simulink model "WeatherAPI"  (R2024b)
settings: Solver=VariableStepAuto  StartTime=0.0  StopTime=86400  FixedStep=0.05  RelTol=1e-3
libraries: spsCurrentMeasurementLib x6, spsGroundLib x6, eePowerMeasurement x6, spsPVArrayLib x6, spsSeriesRLCLoadLib x6, spsVoltageMeasurementLib x6, spspowerguiLib x1
settings Model: Creator=mitphanase  LastModifiedBy=DELL
settings RTWCC: GenCodeOnly=on

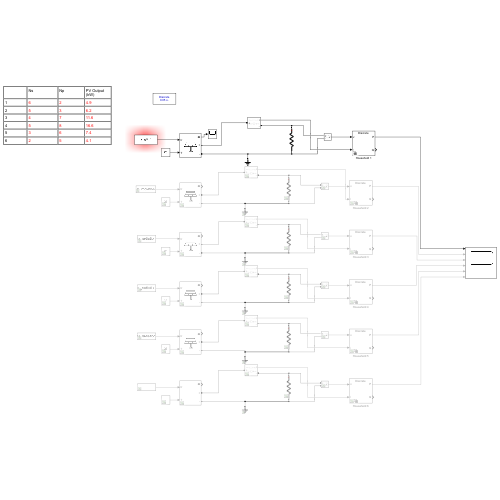
[thumbnail: Simulink's stored preview of the top-level diagram]
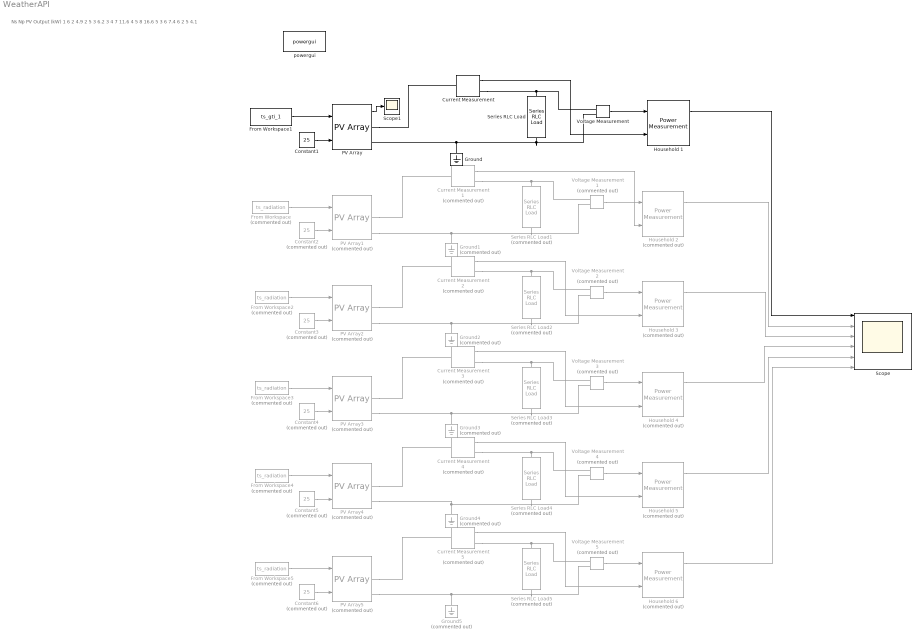
== system WeatherAPI ==
  note: ​
      | Ns
      | Np
      | PV Output (kW)
      |
      | 1
      | 6
      | 2
      | 4.9
      |
      | 2
      | 5
      | 3
      | 6.2
      |
      | 3
      | 4
      | 7
      | 11.6
      |
      | 4
      | 5
      | 8
      | 16.6
      |
      | 5
      | 3
      | 6
      | 7.4
      |
      | 6
      | 2
      | 5
      | 4.1
  Constant1 : Constant  Value=25
  Constant{2..6} (5 alike) : Constant  Commented=on  Value=25
  Current Measurement : spsCurrentMeasurementLib/Current Measurement  PhasorSimulation=off  OutputType=Complex  PSBequivalent=0
  Current Measurement{1..5} (5 alike) : spsCurrentMeasurementLib/Current Measurement  Commented=on  PhasorSimulation=off  OutputType=Complex  PSBequivalent=0
  From Workspace{,2..4} (4 alike) : FromWorkspace  Commented=on  VariableName=ts_radiation  OutDataTypeStr=double
  From Workspace1 : FromWorkspace  VariableName=ts_gti_1  OutDataTypeStr=double
  From Workspace5 : FromWorkspace  Commented=on  VariableName=ts_radiation
  Ground : spsGroundLib/Ground  LConnTagsString=a
  Ground{1..5} (5 alike) : spsGroundLib/Ground  Commented=on  LConnTagsString=a
  Household 1 : eePowerMeasurement/Power Measurement  LabelModeActiveChoice=Discrete  F=60  K=[0]  Ts=60
  "Household 2 " : eePowerMeasurement/Power Measurement  Commented=on  LabelModeActiveChoice=Discrete  F=60  K=[0]  Ts=60
  Household {3..6} (4 alike) : eePowerMeasurement/Power Measurement  Commented=on  LabelModeActiveChoice=Discrete  F=60  K=[0]  Ts=60
  PV Array : spsPVArrayLib/PV Array  Npar=2  Nser=6  PlotType=array @ 1000 W/m2 & specified temperatures  S_vec="[ 1000  500  100 ]"  Temp_C_vec="[ 45 25  ]"  ModuleName=SunPower SPR-415E-WHT-D  PlotWhenSelected=off  Pm=414.801  Ncell=128  Voc=85.3  Isc=6.09  Vm=72.9  Im=5.69  beta_Voc_pc=-0.229  alpha_Isc_pc=0.030706  beta_Voc=-0.19534  alpha_Isc=0.00187  IL=6.0978  I0=7.1698e-13  nI=0.87223  Rsh=419.7781  Rs=0.53711  RobustModel=off  RobustCellTemperature=313.3991  BAL=on  Tc=1e-6  Tfilter=5e-5
  PV Array1 : spsPVArrayLib/PV Array  Commented=on  Npar=3  Nser=5  PlotType=array @ 1000 W/m2 & specified temperatures  S_vec="[ 1000  500  100 ]"  Temp_C_vec="[ 45 25  ]"  ModuleName=SunPower SPR-415E-WHT-D  PlotWhenSelected=off  Pm=414.801  Ncell=128  Voc=85.3  Isc=6.09  Vm=72.9  Im=5.69  beta_Voc_pc=-0.229  alpha_Isc_pc=0.030706  beta_Voc=-0.19534  alpha_Isc=0.00187  IL=6.0978  I0=7.1698e-13  nI=0.87223  Rsh=419.7781  Rs=0.53711  RobustModel=off  RobustCellTemperature=313.3991  BAL=on  Tc=1e-6  Tfilter=5e-5
  PV Array2 : spsPVArrayLib/PV Array  Commented=on  Npar=4  Nser=7  PlotType=array @ 1000 W/m2 & specified temperatures  S_vec="[ 1000  500  100 ]"  Temp_C_vec="[ 45 25  ]"  ModuleName=SunPower SPR-415E-WHT-D  PlotWhenSelected=off  Pm=414.801  Ncell=128  Voc=85.3  Isc=6.09  Vm=72.9  Im=5.69  beta_Voc_pc=-0.229  alpha_Isc_pc=0.030706  beta_Voc=-0.19534  alpha_Isc=0.00187  IL=6.0978  I0=7.1698e-13  nI=0.87223  Rsh=419.7781  Rs=0.53711  RobustModel=off  RobustCellTemperature=313.3991  BAL=on  Tc=1e-6  Tfilter=5e-5
  PV Array3 : spsPVArrayLib/PV Array  Commented=on  Npar=6  Nser=7  PlotType=array @ 1000 W/m2 & specified temperatures  S_vec="[ 1000  500  100 ]"  Temp_C_vec="[ 45 25  ]"  ModuleName=SunPower SPR-415E-WHT-D  PlotWhenSelected=off  Pm=414.801  Ncell=128  Voc=85.3  Isc=6.09  Vm=72.9  Im=5.69  beta_Voc_pc=-0.229  alpha_Isc_pc=0.030706  beta_Voc=-0.19534  alpha_Isc=0.00187  IL=6.0978  I0=7.1698e-13  nI=0.87223  Rsh=419.7781  Rs=0.53711  RobustModel=off  RobustCellTemperature=313.3991  BAL=on  Tc=1e-6  Tfilter=5e-5
  PV Array4 : spsPVArrayLib/PV Array  Commented=on  Npar=3  Nser=6  PlotType=array @ 1000 W/m2 & specified temperatures  S_vec="[ 1000  500  100 ]"  Temp_C_vec="[ 45 25  ]"  ModuleName=SunPower SPR-415E-WHT-D  PlotWhenSelected=off  Pm=414.801  Ncell=128  Voc=85.3  Isc=6.09  Vm=72.9  Im=5.69  beta_Voc_pc=-0.229  alpha_Isc_pc=0.030706  beta_Voc=-0.19534  alpha_Isc=0.00187  IL=6.0978  I0=7.1698e-13  nI=0.87223  Rsh=419.7781  Rs=0.53711  RobustModel=off  RobustCellTemperature=313.3991  BAL=on  Tc=1e-6  Tfilter=5e-5
  PV Array5 : spsPVArrayLib/PV Array  Commented=on  Npar=2  Nser=5  PlotType=array @ 1000 W/m2 & specified temperatures  S_vec="[ 1000  500  100 ]"  Temp_C_vec="[ 45 25  ]"  ModuleName=SunPower SPR-415E-WHT-D  PlotWhenSelected=off  Pm=414.801  Ncell=128  Voc=85.3  Isc=6.09  Vm=72.9  Im=5.69  beta_Voc_pc=-0.229  alpha_Isc_pc=0.030706  beta_Voc=-0.19534  alpha_Isc=0.00187  IL=6.0978  I0=7.1698e-13  nI=0.87223  Rsh=419.7781  Rs=0.53711  RobustModel=off  RobustCellTemperature=313.3991  BAL=on  Tc=1e-6  Tfilter=5e-5
  Scope : Scope  NumInputPorts=6
  Scope1 : Scope
  Series RLC Load : spsSeriesRLCLoadLib/Series RLC Load  LConnTagsString=a  RConnTagsString=__new0  NominalVoltage=400  NominalFrequency=0.0000001  ActivePower=2000  InductivePower=0  CapacitivePower=0  Setx0=off  InitialVoltage=0  SetiL0=off  InitialCurrent=0  Measurements=Branch voltage and current  LoadType=constant I
  Series RLC Load1 : spsSeriesRLCLoadLib/Series RLC Load  Commented=on  LConnTagsString=a  RConnTagsString=__new0  NominalVoltage=400  NominalFrequency=0.0000001  ActivePower=3500  InductivePower=0  CapacitivePower=0  Setx0=off  InitialVoltage=0  SetiL0=off  InitialCurrent=0  Measurements=Branch voltage and current  LoadType=constant I
  Series RLC Load2 : spsSeriesRLCLoadLib/Series RLC Load  Commented=on  LConnTagsString=a  RConnTagsString=__new0  NominalVoltage=400  NominalFrequency=0.0000001  ActivePower=6000  InductivePower=0  CapacitivePower=0  Setx0=off  InitialVoltage=0  SetiL0=off  InitialCurrent=0  Measurements=Branch voltage and current  LoadType=constant I
  Series RLC Load3 : spsSeriesRLCLoadLib/Series RLC Load  Commented=on  LConnTagsString=a  RConnTagsString=__new0  NominalVoltage=400  NominalFrequency=0.0000001  ActivePower=10000  InductivePower=0  CapacitivePower=0  Setx0=off  InitialVoltage=0  SetiL0=off  InitialCurrent=0  Measurements=Branch voltage and current  LoadType=constant I
  Series RLC Load4 : spsSeriesRLCLoadLib/Series RLC Load  Commented=on  LConnTagsString=a  RConnTagsString=__new0  NominalVoltage=400  NominalFrequency=0.0000001  ActivePower=5000  InductivePower=0  CapacitivePower=0  Setx0=off  InitialVoltage=0  SetiL0=off  InitialCurrent=0  Measurements=Branch voltage and current  LoadType=constant I
  Series RLC Load5 : spsSeriesRLCLoadLib/Series RLC Load  Commented=on  LConnTagsString=a  RConnTagsString=__new0  NominalVoltage=400  NominalFrequency=0.0000001  ActivePower=4000  InductivePower=0  CapacitivePower=0  Setx0=off  InitialVoltage=0  SetiL0=off  InitialCurrent=0  Measurements=Branch voltage and current  LoadType=constant I
  Voltage Measurement : spsVoltageMeasurementLib/Voltage Measurement  PhasorSimulation=off  OutputType=Complex  PSBequivalent=0
  Voltage Measurement{1..5} (5 alike) : spsVoltageMeasurementLib/Voltage Measurement  Commented=on  PhasorSimulation=off  OutputType=Complex  PSBequivalent=0
  powergui : spspowerguiLib/powergui  Priority=1  SimulationMode=Discrete  SampleTime=0.05  frequency=60  Iterations=50  frequencyindice=0  Pbase=100e6  ErrMax=1e-4  UnitsV=kV  UnitsW=MW  buscounter=0  FunctionMessages=off  echomessages=off  EnableUseOfTLC=off  CurrentSourceSwitches=off  DisableSnubberDevices=off  DisableRonSwitches=off  DisableVfSwitches=off  DisplayEquations=off  AutomaticDiscreteSolvers=off  SolverType=Tustin/Backward Euler (TBE)  Interpol=off  ExternalGateDelay=off  methode=off  Ts=100  x0status=blocks  SPID=on  SwTol=0  HookPort=off  NonlinearTolerance=1e-4  nMaxIteration=100  ContinueOnMaxIteration=off  RestoreLinks=warning  ResistiveCurrentMeasurement=off  Frange=[0:2:500]  Ylog=off  Xlog=on  ShowGrid=off  save=off  variable=ZData  structure=0  ZoomFFT=off  StartTime=0.0  cycles=1  DisplayStyle=1  fundamental=60  FreqAxis=off  MaxFrequency=1000  frequencyindicesteady=1  RmsSteady=1  display=off
  wires:
  Constant1/1 -> PV Array/2
  From Workspace1/1 -> PV Array/1
  Current Measurement/1 -> Household 1/2
  Voltage Measurement/1 -> Household 1/1
  From Workspace/1 -> PV Array1/1
  From Workspace2/1 -> PV Array2/1
  From Workspace3/1 -> PV Array3/1
  From Workspace4/1 -> PV Array4/1
  From Workspace5/1 -> PV Array5/1
  Constant2/1 -> PV Array1/2
  Constant3/1 -> PV Array2/2
  Constant4/1 -> PV Array3/2
  Constant5/1 -> PV Array4/2
  Constant6/1 -> PV Array5/2
  Current Measurement1/1 -> "Household 2 "/2
  Voltage Measurement1/1 -> "Household 2 "/1
  Current Measurement2/1 -> Household 3/2
  Voltage Measurement2/1 -> Household 3/1
  Current Measurement3/1 -> Household 4/2
  Voltage Measurement3/1 -> Household 4/1
  Current Measurement4/1 -> Household 5/2
  Voltage Measurement4/1 -> Household 5/1
  Current Measurement5/1 -> Household 6/2
  Voltage Measurement5/1 -> Household 6/1
  Household 1/1 -> Scope/1
  "Household 2 "/1 -> Scope/2
  Household 3/1 -> Scope/3
  Household 4/1 -> Scope/4
  Household 5/1 -> Scope/5
  Household 6/1 -> Scope/6
  PV Array/1 -> Scope1/1
  connections:
  Series RLC Load/RConn1 -- Ground/LConn1 -- PV Array/RConn2 -- Voltage Measurement/LConn2
  PV Array/RConn1 -- Current Measurement/LConn1
  Current Measurement/RConn1 -- Voltage Measurement/LConn1 -- Series RLC Load/LConn1
  Ground1/LConn1 -- PV Array1/RConn2 -- Voltage Measurement1/LConn2 -- Series RLC Load1/RConn1
  Current Measurement1/RConn1 -- Voltage Measurement1/LConn1 -- Series RLC Load1/LConn1
  PV Array1/RConn1 -- Current Measurement1/LConn1
  Ground2/LConn1 -- PV Array2/RConn2 -- Voltage Measurement2/LConn2 -- Series RLC Load2/RConn1
  Current Measurement2/RConn1 -- Voltage Measurement2/LConn1 -- Series RLC Load2/LConn1
  PV Array2/RConn1 -- Current Measurement2/LConn1
  Ground3/LConn1 -- PV Array3/RConn2 -- Voltage Measurement3/LConn2 -- Series RLC Load3/RConn1
  Current Measurement3/RConn1 -- Voltage Measurement3/LConn1 -- Series RLC Load3/LConn1
  PV Array3/RConn1 -- Current Measurement3/LConn1
  Ground4/LConn1 -- PV Array4/RConn2 -- Voltage Measurement4/LConn2 -- Series RLC Load4/RConn1
  Current Measurement4/RConn1 -- Voltage Measurement4/LConn1 -- Series RLC Load4/LConn1
  PV Array4/RConn1 -- Current Measurement4/LConn1
  Ground5/LConn1 -- PV Array5/RConn2 -- Voltage Measurement5/LConn2 -- Series RLC Load5/RConn1
  Current Measurement5/RConn1 -- Voltage Measurement5/LConn1 -- Series RLC Load5/LConn1
  PV Array5/RConn1 -- Current Measurement5/LConn1
